simulink library "slib_spectrum_analyser"  (R2020a)
settings: Solver=VariableStepAuto  StartTime=0.0  StopTime=10.0  RelTol=1e-3
libraries: hdlsllib x104, simulink x49, dsphdlxfrm x5, $bdroot x5
(part 3 of 3)

== system slib_spectrum_analyser/SSR Subset Converter/SSR Serializer Real/Vector to SSR ==
  Vector : Inport
  Bit Concat : hdlsllib/Logic and Bit Operations/Bit Concat  numInputs=8
  Selector0 : Selector  InputPortWidth=8  IndexOptions=Index vector (dialog)  Indices=8  OutputSizes=1
  Selector1 : Selector  InputPortWidth=8  IndexOptions=Index vector (dialog)  Indices=7  OutputSizes=1
  Selector2 : Selector  InputPortWidth=8  IndexOptions=Index vector (dialog)  Indices=6  OutputSizes=1
  Selector3 : Selector  InputPortWidth=8  IndexOptions=Index vector (dialog)  Indices=5  OutputSizes=1
  Selector4 : Selector  InputPortWidth=8  IndexOptions=Index vector (dialog)  Indices=4  OutputSizes=1
  Selector5 : Selector  InputPortWidth=8  IndexOptions=Index vector (dialog)  Indices=3  OutputSizes=1
  Selector6 : Selector  InputPortWidth=8  IndexOptions=Index vector (dialog)  Indices=2  OutputSizes=1
  Selector7 : Selector  InputPortWidth=8  IndexOptions=Index vector (dialog)  Indices=1  OutputSizes=1
  SSR : Outport
  wires:
  Bit Concat/1 -> SSR/1
  Vector/1 -> Selector6/1, Selector7/1, Selector5/1, Selector4/1, Selector3/1, Selector2/1, Selector1/1, Selector0/1
  Selector0/1 -> Bit Concat/1
  Selector1/1 -> Bit Concat/2
  Selector2/1 -> Bit Concat/3
  Selector3/1 -> Bit Concat/4
  Selector4/1 -> Bit Concat/5
  Selector5/1 -> Bit Concat/6
  Selector6/1 -> Bit Concat/7
  Selector7/1 -> Bit Concat/8

== matlab function slib_spectrum_analyser/Direct Memory Access/Direct Memory Access/DDR Communication/Write Controller ==
  data: valid input; count input; push output boolean; pop output; length input; enable input; start input boolean; wr_complete input; wr_ready input; wr_len output; buffer output; state output; empty input; debug_count output
function [push, pop, wr_len, buffer, state, debug_count] = ddr_write_control(valid, count, length, enable, start, wr_complete, wr_ready, empty)

% Create persistent variables (registers)
persistent burst_count;
persistent time_count;
persistent current_state;
persistent buffer_pointer;

if(isempty(burst_count))
    burst_count = fi(0, 0, 16, 0);
end

if(isempty(time_count))
    time_count = fi(0, 0, 32, 0);
end

if(isempty(current_state))
    current_state = fi(0, 0, 4, 0);
end

if(isempty(buffer_pointer))
    buffer_pointer = fi(0, 0, 2, 0);
end

% FSM States
IDLE  = fi(0, 0, 4, 0);
START = fi(1, 0, 4, 0);
COUNT = fi(2, 0, 4, 0);
WAIT  = fi(4, 0, 4, 0);

switch current_state
    case IDLE
        push = false;
        pop = wr_ready;
        wr_len = length;
        buffer = buffer_pointer;
        state = current_state;
        debug_count = burst_count;
        
        burst_count = fi(0, 0, 16, 0);
        
        if enable && time_count >= count
            current_state = START;
            time_count = fi(0, 0, 32, 0);
        else
            current_state = IDLE;
            if time_count < count
                time_count = fi(time_count + 1, 0, 32, 0);
            end
        end
        
    case START
        pop = false;
        wr_len = length;
        buffer = buffer_pointer;
        state = current_state;
        debug_count = burst_count;
        
        if ~enable
            push = false;
            burst_count = fi(0, 0, 16, 0);
            current_state = IDLE;
        else
            if start && valid
                push = true;
                burst_count = fi(burst_count + 1, 0, 16, 0);
                current_state = COUNT;
            else
                push = false;
                burst_count = fi(0, 0, 16, 0);
                current_state = START;
            end
        end            
        
    case COUNT
        pop = false;
        wr_len = length;
        buffer = buffer_pointer;
        state = current_state;
        debug_count = burst_count;
        
        if valid
            push = true;
            burst_count = fi(burst_count + 1, 0, 16, 0);
        else
            push = false;
        end
        
        if burst_count >= length
            current_state = WAIT;
            if buffer_pointer > fi(1, 0, 2, 0)
                buffer_pointer = fi(0, 0, 2, 0);
            else
            	buffer_pointer = fi(buffer_pointer+1, 0, 2, 0);
            end
        else
            current_state = COUNT;
        end
        
    case WAIT
        push = false;
        pop = wr_ready;
        wr_len = length;
        buffer = buffer_pointer;
        state = current_state;
        debug_count = burst_count;
        
        burst_count = fi(0, 0, 16, 0);
        
        if empty && wr_complete
            current_state = IDLE;
        else
            current_state = WAIT;
        end
        
    otherwise
        push = false;
        pop = wr_ready;
        wr_len = length;
        buffer = buffer_pointer;
        state = current_state;
        debug_count = burst_count;
        
        burst_count = fi(0, 0, 16, 0);
        
        current_state = IDLE;
        
end

== matlab function slib_spectrum_analyser/Preprocessing Window/Direct Memory Access/DDR Read Controller ==
  data: valid_out output boolean; count_out output; ready_out output boolean; length_in input; address input; start input boolean; rd_aready input; rd_dvalid input; rd_addr output uint32; rd_len output; rd_avalid output
function [valid_out,count_out,ready_out,rd_addr,rd_len,rd_avalid] = ddr_read_control(length_in, address, start, rd_aready, rd_dvalid)

% Create persistent variables (registers)
persistent burst_stop
if(isempty(burst_stop))
    burst_stop = uint16(0);
end
persistent burst_count;
if(isempty(burst_count))
    burst_count = uint16(0);
end
persistent rstate;
if isempty(rstate)
    rstate = fi(0, 0, 4, 0);
end


% State Memory Encoding
IDLE             = fi(1, 0, 4, 0);
READ_BURST_START = fi(2, 0, 4, 0);
DATA_COUNT       = fi(4, 0, 4, 0);

% Read control state machine
switch (rstate)
    case IDLE
        % output to AXI4 Master
        rd_addr = address;
        rd_len = uint16(0);
        rd_avalid = false;
        
        % output to DUT
        valid_out = false;
        ready_out = true;
        count_out = uint16(0);
        
        % State vars
        burst_count = uint16(0);
        burst_stop = uint16(length_in);
        
        if rd_aready && start
            rstate(:) = READ_BURST_START;
        end
        
    case READ_BURST_START
        % output to AXI4 Master
        rd_addr = address;
        rd_len = uint16(burst_stop);
        rd_avalid = true;
        
        % output to DUT
        valid_out = false;
        count_out = uint16(0);
        ready_out = false;
        
        rstate(:) = DATA_COUNT;
        
    case DATA_COUNT
        % output to AXI4 Master
        rd_addr = address;
        rd_len = uint16(burst_stop);
        rd_avalid = false;
        
        % output to DUT
        valid_out = rd_dvalid;
        count_out = uint16(burst_count);
        ready_out = false;
        
        % State vars
        if ( rd_dvalid )
            burst_count = uint16(burst_count + 1);
        end
        
        if ( burst_count == burst_stop )
            rstate(:) = IDLE;
        else
            rstate(:) = DATA_COUNT;
        end
        
    otherwise
        % output to AXI4 Master
        rd_addr = uint32(0);
        rd_len = uint16(0);
        rd_avalid = false;
        
        % output to DUT
        valid_out = false;
        count_out = uint16(0);
        ready_out = false;
        
        rstate(:) = IDLE;
end

end
